simulink model "RotatingMasses_Template"  (R2019b)
settings: Solver=ode1  StartTime=0.0  StopTime=110  FixedStep=0.002  RelTol=1e-3  EnableMultiTasking=on
PostLoadFcn:
  | qc_set_target_type(getConfigSet(bdroot, 'QUARC Default Target Configuration'));
values from neighbouring files (symbols this model uses):
  data = dataset_struct    [create_data.m]    (also in data_loader.m = [])
  deg_to_rad = pi/180    (= 0.0174532925199)    [sensors_parameters.m]
  experiment = merge( experiment, experiment2 )    [blackbox_est.m]    (also in experiment_handler.m = obj.experiments{idx_exp}; guided_script.m = e_h.experiments{40}; test_controllori.m = e_h.load_experiment)
  pulse_to_rad = 2*pi/pulse_per_rev_encoder    (= 0.00153398078789)    [sensors_parameters.m]
  V_th = V_max*1    [sensors_parameters.m]
  Vmin_pot = -4.8924    [sensors_parameters.m]
  volt_to_deg_potentiometer = 352/(Vmax_pot-Vmin_pot)    (= 36.7512711555)    [sensors_parameters.m]
undefined symbols (not defined in the file or in its folder): controller, HIL, qc_get_step_size
libraries: simulink x43, cstblocks x15, quarc_library x5
(part 3 of 3)

== matlab function RotatingMasses_Template/Controllers/C1: speed loop  mass 1/Reference/MATLAB Function ==
  data: i_t input; step output; s_a input; t input
function step = multistep(i_t, s_a, t)

% it is assumed i_t is sorted!

% find the first time step that is greater than actual time. 
step = 0;
for idx = 1:length(i_t) 
    if i_t(idx) <= t
        step = s_a(idx);
    end
end

== matlab function RotatingMasses_Template/Controllers/C2: position loop mass 1/Reference/MATLAB Function ==
  data: i_t input; step output; s_a input; t input
function step = multistep(i_t, s_a, t)

% it is assumed i_t is sorted!

% find the first time step that is greater than actual time. 
step = 0;
for idx = 1:length(i_t) 
    if i_t(idx) <= t
        step = s_a(idx);
    end
end

== matlab function RotatingMasses_Template/Controllers/C3: speed loop  mass 2/Reference/MATLAB Function ==
  data: i_t input; step output; s_a input; t input
function step = multistep(i_t, s_a, t)

% it is assumed i_t is sorted!

% find the first time step that is greater than actual time. 
step = 0;
for idx = 1:length(i_t) 
    if i_t(idx) <= t
        step = s_a(idx);
    end
end

== matlab function RotatingMasses_Template/Controllers/C4: position loop mass 2/Reference/MATLAB Function ==
  data: i_t input; step output; s_a input; t input
function step = multistep(i_t, s_a, t)

% it is assumed i_t is sorted!

% find the first time step that is greater than actual time. 
step = 0;
for idx = 1:length(i_t) 
    if i_t(idx) <= t
        step = s_a(idx);
    end
end

== matlab function RotatingMasses_Template/Controllers/C5: speed loop  mass 1/Reference/MATLAB Function ==
  data: i_t input; step output; s_a input; t input
function step = multistep(i_t, s_a, t)

% it is assumed i_t is sorted!

% find the first time step that is greater than actual time. 
step = 0;
for idx = 1:length(i_t) 
    if i_t(idx) <= t
        step = s_a(idx);
    end
end

== matlab function RotatingMasses_Template/Controllers/C6: speed loop  mass 2/Reference/MATLAB Function ==
  data: i_t input; step output; s_a input; t input
function step = multistep(i_t, s_a, t)

% it is assumed i_t is sorted!

% find the first time step that is greater than actual time. 
step = 0;
for idx = 1:length(i_t) 
    if i_t(idx) <= t
        step = s_a(idx);
    end
end

== matlab function RotatingMasses_Template/Controllers/C7: position loop  mass 1/Reference/MATLAB Function ==
  data: i_t input; step output; s_a input; t input
function step = multistep(i_t, s_a, t)

% it is assumed i_t is sorted!

% find the first time step that is greater than actual time. 
step = 0;
for idx = 1:length(i_t) 
    if i_t(idx) <= t
        step = s_a(idx);
    end
end

== matlab function RotatingMasses_Template/Controllers/C14: Pole placement + red observer 1dof, pos1/Reference/MATLAB Function ==
  data: i_t input; step output; s_a input; t input
function step = multistep(i_t, s_a, t)

% it is assumed i_t is sorted!

% find the first time step that is greater than actual time. 
step = 0;
for idx = 1:length(i_t) 
    if i_t(idx) <= t
        step = s_a(idx);
    end
end

== matlab function RotatingMasses_Template/Controllers/C15: Pole placement + observer 2dof, speed1/Reference/MATLAB Function ==
  data: i_t input; step output; s_a input; t input
function step = multistep(i_t, s_a, t)

% it is assumed i_t is sorted!

% find the first time step that is greater than actual time. 
step = 0;
for idx = 1:length(i_t) 
    if i_t(idx) <= t
        step = s_a(idx);
    end
end

== matlab function RotatingMasses_Template/Controllers/C16: Pole placement + observer 2dof, pos1/Reference/MATLAB Function ==
  data: i_t input; step output; s_a input; t input
function step = multistep(i_t, s_a, t)

% it is assumed i_t is sorted!

% find the first time step that is greater than actual time. 
step = 0;
for idx = 1:length(i_t) 
    if i_t(idx) <= t
        step = s_a(idx);
    end
end

== matlab function RotatingMasses_Template/Controllers/C13: Pole placement + red observer 1dof, speed1/Reference/MATLAB Function ==
  data: i_t input; step output; s_a input; t input
function step = multistep(i_t, s_a, t)

% it is assumed i_t is sorted!

% find the first time step that is greater than actual time. 
step = 0;
for idx = 1:length(i_t) 
    if i_t(idx) <= t
        step = s_a(idx);
    end
end

== matlab function RotatingMasses_Template/Controllers/C8: position loop  mass 2/Reference/MATLAB Function ==
  data: i_t input; step output; s_a input; t input
function step = multistep(i_t, s_a, t)

% it is assumed i_t is sorted!

% find the first time step that is greater than actual time. 
step = 0;
for idx = 1:length(i_t) 
    if i_t(idx) <= t
        step = s_a(idx);
    end
end

== matlab function RotatingMasses_Template/Controllers/Reference/MATLAB Function ==
  data: i_t input; step output; s_a input; t input
function step = multistep(i_t, s_a, t)

% it is assumed i_t is sorted!

% find the first time step that is greater than actual time. 
step = 0;
for idx = 1:length(i_t) 
    if i_t(idx) <= t
        step = s_a(idx);
    end
end

== matlab function RotatingMasses_Template/Controllers/1dof Observers/MATLAB Function1 ==
  data: u input; y output
function y = fcn(u)
persistent oldu
if isempty(oldu) 
    oldu = u;
end
y = oldu;

== matlab function RotatingMasses_Template/Controllers/2dof Observers/MATLAB Function1 ==
  data: u input; y output
function y = fcn(u)
persistent oldu
if isempty(oldu) 
    oldu = u;
end
y = oldu;

== matlab function RotatingMasses_Template/potentiometer/Starting position ==
  data: u input; y output
function y = fcn(u)
persistent oldu
if isempty(oldu) 
    oldu = u;
end
y = oldu;

== matlab function RotatingMasses_Template/Controllers/C9: Pole placement + observer 1dof, speed/Reference/MATLAB Function ==
  data: i_t input; step output; s_a input; t input
function step = multistep(i_t, s_a, t)

% it is assumed i_t is sorted!

% find the first time step that is greater than actual time. 
step = 0;
for idx = 1:length(i_t) 
    if i_t(idx) <= t
        step = s_a(idx);
    end
end

== matlab function RotatingMasses_Template/Controllers/C10: Pole placement + observer 1dof, pos/Reference/MATLAB Function ==
  data: i_t input; step output; s_a input; t input
function step = multistep(i_t, s_a, t)

% it is assumed i_t is sorted!

% find the first time step that is greater than actual time. 
step = 0;
for idx = 1:length(i_t) 
    if i_t(idx) <= t
        step = s_a(idx);
    end
end

== matlab function RotatingMasses_Template/Controllers/C11: Pole placement + observer 2dof, speed/Reference/MATLAB Function ==
  data: i_t input; step output; s_a input; t input
function step = multistep(i_t, s_a, t)

% it is assumed i_t is sorted!

% find the first time step that is greater than actual time. 
step = 0;
for idx = 1:length(i_t) 
    if i_t(idx) <= t
        step = s_a(idx);
    end
end

== matlab function RotatingMasses_Template/Controllers/C12: Pole placement + observer 2dof, pos/Reference/MATLAB Function ==
  data: i_t input; step output; s_a input; t input
function step = multistep(i_t, s_a, t)

% it is assumed i_t is sorted!

% find the first time step that is greater than actual time. 
step = 0;
for idx = 1:length(i_t) 
    if i_t(idx) <= t
        step = s_a(idx);
    end
end
